simulink model "mdlref_counter_paramargs"  (Simulink 6.0)
settings: Solver=FixedStepDiscrete  StartTime=0.0  StopTime=10.0  FixedStep=Auto  RelTol=1e-3
model workspace: external: MAT-File (data not in the file)
values from neighbouring files (symbols this model uses):
  lower_saturation_limit = 0    [mdlref_counter_paramargs_init.mat]
  upper_saturation_limit = 1    [mdlref_counter_paramargs_init.mat]
settings Model: Creator=The MathWorks Inc.  LastModifiedBy=batserve  ExtModeAutoUpdateStatusClock=off  ProdHWDeviceType=Specified
settings DataIOCC: SaveFormat=StructureWithTime  SignalLoggingName=logsOut
settings OptimizationCC: InlineParams=on
settings DebuggingCC: CheckExecutionContextPreStartOutputMsg=on  CheckExecutionContextRuntimeOutputMsg=on  SignalResolutionControl=UseLocalSettings  SolverPrmCheckMsg=none
settings HardwareCC: ProdHWDeviceType=Specified  TargetHWDeviceType=32-bit Generic  ProdEqTarget=off
settings ModelReferenceCC: UpdateModelReferenceTargets=IfOutOfDate  CheckModelReferenceTargetMessage=none
settings RTWCC: GenerateReport=on  ProcessScript=grt_make_rtw_hook  LaunchReport=on

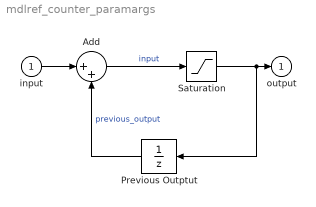
== system mdlref_counter_paramargs ==
  " input" : Inport  Port=1  LatchInput=off
  Add : Sum  Inputs=|++  OutScaling=2^-10
  Previous Outptut : UnitDelay  Orientation=left  SampleTime=-1
  Saturation : Saturate  UpperLimit=upper_saturation_limit  LowerLimit=lower_saturation_limit
  output : Outport
  wires:
  Previous Outptut/1 -> Add/2  "previous_output"
  " input"/1 -> Add/1
  Add/1 -> Saturation/1  "input"
  Saturation/1 -> output/1, Previous Outptut/1
